simulink model "sampleModel1670"  (R2023a)
settings: Solver=VariableStepAuto  StartTime=0.0  StopTime=10.0  RelTol=1e-3
libraries: hdlsllib x7, simulink x1
settings Model: Creator=user1  LastModifiedBy=user1

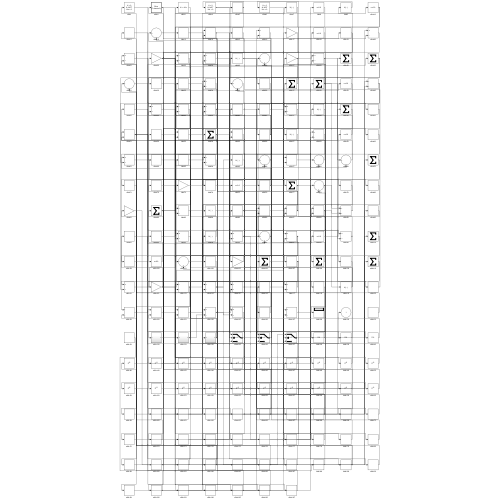
[thumbnail: Simulink's stored preview of the top-level diagram]
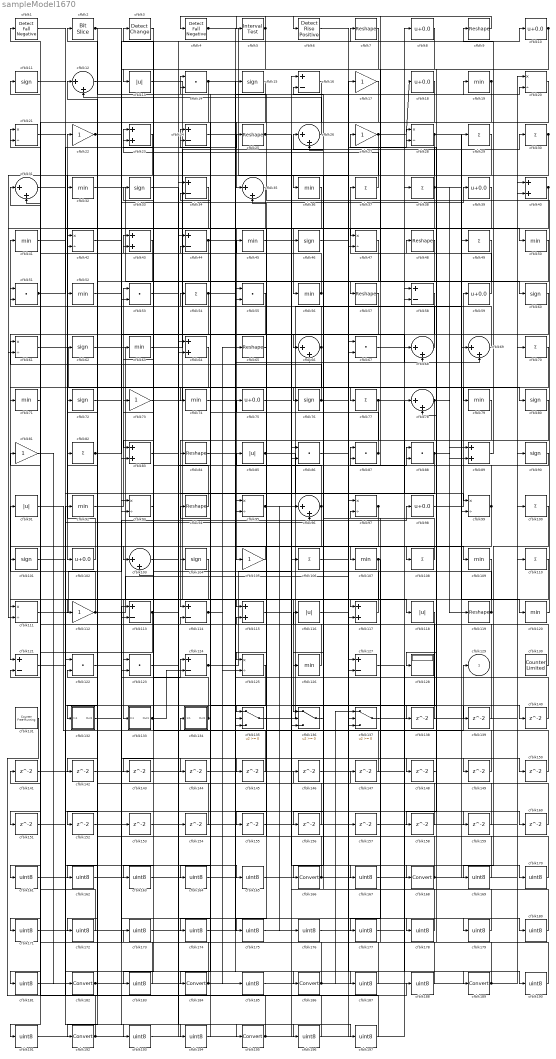
== system sampleModel1670 ==
  cfblk1 : hdlsllib/Logic and Bit Operations/Detect Fall Negative  vinit=0  OutDataTypeStr=boolean
  cfblk{8,10,18,39,59,75,98,102} (8 alike) : Bias  Bias=0.0  SaturateOnIntegerOverflow=off
  cfblk{29..30,37..38,49,54,70,77,82,100,106,108,110} (13 alike) : Sum  Inputs=+
  cfblk{11,15,33,46,60,62,72,76,80,90,101,104} (12 alike) : Signum
  cfblk{12,26,31,35,66,68..69,78,96,103} (10 alike) : Sum  Inputs=|++
  cfblk{17,22,27,73,81,105,112} (7 alike) : Gain
  cfblk{19,32,36,41,45,50,52,56,63,71,74,79,92,107,109,120,126} (17 alike) : MinMax
  cfblk{20..21,28,42,47,61,93,95,97,99,111,125} (12 alike) : Product  Inputs=*/  RndMeth=Zero  SaturateOnIntegerOverflow=on
  cfblk{16,24,34,44,58,113..114,121,124,127} (10 alike) : Sum  Inputs=+-
  cfblk{23,40,43,64,83,89,115,117} (8 alike) : Sum
  cfblk{13,85,91,116,118} (5 alike) : Abs  SaturateOnIntegerOverflow=off
  cfblk{7,9,25,48,57,65,84,94,119} (9 alike) : Reshape
  cfblk{14,51,53,55,67,86..88,122..123} (10 alike) : DotProduct  OutDataTypeStr=Inherit: Inherit via internal rule
  cfblk128 : Display
  cfblk130 : hdlsllib/Sources/Counter Limited  uplimit=7  tsamp=-1
  cfblk131 : hdlsllib/Sources/Counter Free-Running  NumBits=16  tsamp=-1
  cfblk132 : Subsystem
      settings: LibrarySourceBlock=|
      | hdlsllib/Ports &
      | Subsystems/Subsystem
  cfblk133 : Subsystem
      settings: LibrarySourceBlock=|
      | hdlsllib/Ports &
      | Subsystems/Subsystem
  cfblk134 : Subsystem
      settings: LibrarySourceBlock=|
      | hdlsllib/Ports &
      | Subsystems/Subsystem
  cfblk135 : Switch  SaturateOnIntegerOverflow=off  InputSameDT=off
  cfblk136 : Switch  SaturateOnIntegerOverflow=off  InputSameDT=off
  cfblk137 : Switch  SaturateOnIntegerOverflow=off  InputSameDT=off
  cfblk{138..160} (23 alike) : Delay  SampleTime=1
  cfblk{161..165,167,169..181,183,185,187..188,190..191,193..194,196..197} (29 alike) : DataTypeConversion  OutDataTypeStr=uint8  SaturateOnIntegerOverflow=off  RndMeth=Floor
  cfblk{166,168,182,184,186,189,192,195} (8 alike) : DataTypeConversion  SaturateOnIntegerOverflow=off  RndMeth=Floor
  cfblk2 : hdlsllib/Logic and Bit Operations/Bit Slice  lidx=7  ridx=0
  cfblk3 : simulink/Logic and Bit Operations/Detect Change  vinit=0  OutDataTypeStr=boolean
      settings: LibrarySourceBlock=|
      | hdlsllib/Logic and Bit
      | Operations/Detect
      | Change
  cfblk4 : hdlsllib/Logic and Bit Operations/Detect Fall Negative  vinit=0  OutDataTypeStr=boolean
  cfblk5 : hdlsllib/Logic and Bit Operations/Interval Test  IntervalClosedRight=on  uplimit=0.5  IntervalClosedLeft=on  lowlimit=-0.5  OutDataTypeStr=boolean
  cfblk6 : hdlsllib/Logic and Bit Operations/Detect Rise Positive  vinit=0  OutDataTypeStr=boolean
  cfblk129 : Outport  VectorParamsAs1DForOutWhenUnconnected=off
  wires:
  cfblk114/1 -> cfblk65/1, cfblk185/1
  cfblk68/1 -> cfblk22/1
  cfblk77/1 -> cfblk114/1, cfblk99/1
  cfblk7/1 -> cfblk13/1
  cfblk38/1 -> cfblk6/1, cfblk119/1, cfblk36/1, cfblk60/1, cfblk156/1
  cfblk120/1 -> cfblk2/1
  cfblk85/1 -> cfblk137/2, cfblk167/1
  cfblk49/1 -> cfblk121/1
  cfblk23/1 -> cfblk102/1
  cfblk92/1 -> cfblk53/1
  cfblk62/1 -> cfblk118/1
  cfblk63/1 -> cfblk30/1
  cfblk135/1 -> cfblk88/1
  cfblk35/1 -> cfblk105/1
  cfblk13/1 -> cfblk117/1
  cfblk20/1 -> cfblk42/1
  cfblk34/1 -> cfblk192/1
  cfblk39/1 -> cfblk56/1
  cfblk61/1 -> cfblk80/1
  cfblk48/1 -> cfblk53/2
  cfblk102/1 -> cfblk52/1
  cfblk47/1 -> cfblk132/1(In1)
  cfblk122/1 -> cfblk195/1
  cfblk110/1 -> cfblk184/1
  cfblk119/1 -> cfblk85/1, cfblk33/1
  cfblk73/1 -> cfblk77/1
  cfblk91/1 -> cfblk129/1
  cfblk98/1 -> cfblk59/1
  cfblk3/1 -> cfblk83/1
  cfblk15/1 -> cfblk35/1
  cfblk124/1 -> cfblk46/1, cfblk125/2
  cfblk95/1 -> cfblk29/1, cfblk176/1
  cfblk97/1 -> cfblk151/1, cfblk152/1
  cfblk54/1 -> cfblk71/1, cfblk137/3
  cfblk78/1 -> cfblk84/1, cfblk89/1
  cfblk44/1 -> cfblk62/1, cfblk69/2, cfblk24/1
  cfblk130/1 -> cfblk54/1
  cfblk113/1 -> cfblk87/1, cfblk171/1
  cfblk51/1 -> cfblk25/1, cfblk93/2, cfblk21/2, cfblk159/1
  cfblk31/1 -> cfblk186/1
  cfblk84/1 -> cfblk19/1
  cfblk101/1 -> cfblk115/1
  cfblk99/1 -> cfblk27/1, cfblk135/3
  cfblk65/1 -> cfblk125/1
  cfblk105/1 -> cfblk103/1
  cfblk5/1 -> cfblk4/1, cfblk163/1
  cfblk69/1 -> cfblk41/1
  cfblk111/1 -> cfblk98/1
  cfblk87/1 -> cfblk14/1, cfblk14/2
  cfblk29/1 -> cfblk76/1
  cfblk112/1 -> cfblk91/1, cfblk47/2, cfblk179/1
  cfblk107/1 -> cfblk133/1(In1), cfblk177/1
  cfblk12/1 -> cfblk79/1
  cfblk75/1 -> cfblk109/1
  cfblk66/1 -> cfblk83/2, cfblk23/2
  cfblk2/1 -> cfblk68/2, cfblk142/1
  cfblk80/1 -> cfblk108/1
  cfblk76/1 -> cfblk20/2, cfblk61/1
  cfblk16/1 -> cfblk101/1
  cfblk82/1 -> cfblk39/1, cfblk10/1
  cfblk96/1 -> cfblk123/1, cfblk75/1
  cfblk27/1 -> cfblk18/1, cfblk61/2
  cfblk53/1 -> cfblk7/1
  cfblk86/1 -> cfblk28/1
  cfblk4/1 -> cfblk97/1, cfblk117/2
  cfblk109/1 -> cfblk136/1
  cfblk123/1 -> cfblk44/1
  cfblk118/1 -> cfblk136/2
  cfblk70/1 -> cfblk166/1
  cfblk28/1 -> cfblk120/1, cfblk135/2
  cfblk30/1 -> cfblk128/1, cfblk32/1
  cfblk74/1 -> cfblk15/1
  cfblk136/1 -> cfblk26/1
  cfblk14/1 -> cfblk107/1, cfblk162/1
  cfblk19/1 -> cfblk74/1, cfblk138/1
  cfblk59/1 -> cfblk37/1
  cfblk126/1 -> cfblk21/1
  cfblk56/1 -> cfblk11/1, cfblk24/2
  cfblk94/1 -> cfblk63/1
  cfblk89/1 -> cfblk9/1
  cfblk43/1 -> cfblk112/1
  cfblk71/1 -> cfblk111/1
  cfblk121/1 -> cfblk92/1
  cfblk9/1 -> cfblk5/1
  cfblk8/1 -> cfblk57/1
  cfblk127/1 -> cfblk189/1
  cfblk50/1 -> cfblk126/1
  cfblk134/1(Out1) -> cfblk3/1, cfblk73/1
  cfblk21/1 -> cfblk47/1
  cfblk10/1 -> cfblk113/2, cfblk158/1
  cfblk37/1 -> cfblk23/1
  cfblk11/1 -> cfblk135/1
  cfblk32/1 -> cfblk69/1
  cfblk22/1 -> cfblk93/1, cfblk99/2, cfblk144/1, cfblk145/1
  cfblk137/1 -> cfblk100/1
  cfblk26/1 -> cfblk12/2
  cfblk108/1 -> cfblk51/1
  cfblk1/1 -> cfblk96/2
  cfblk117/1 -> cfblk16/2
  cfblk81/1 -> cfblk182/1
  cfblk45/1 -> cfblk168/1
  cfblk88/1 -> cfblk104/1, cfblk89/2
  cfblk133/1(Out1) -> cfblk43/1, cfblk124/2
  cfblk67/1 -> cfblk38/1
  cfblk90/1 -> cfblk87/2
  cfblk25/1 -> cfblk50/1, cfblk160/1
  cfblk132/1(Out1) -> cfblk124/1
  cfblk79/1 -> cfblk95/2
  cfblk40/1 -> cfblk66/1, cfblk111/2
  cfblk57/1 -> cfblk67/2
  cfblk138/1 -> cfblk1/1
  cfblk83/1 -> cfblk139/1
  cfblk139/1 -> cfblk78/2
  cfblk115/1 -> cfblk140/1
  cfblk140/1 -> cfblk95/1
  cfblk141/1 -> cfblk123/2
  cfblk142/1 -> cfblk96/1
  cfblk93/1 -> cfblk143/1
  cfblk144/1 -> cfblk68/1
  cfblk145/1 -> cfblk103/2
  cfblk147/1 -> cfblk43/2
  cfblk6/1 -> cfblk148/1
  cfblk148/1 -> cfblk28/2
  cfblk116/1 -> cfblk149/1
  cfblk149/1 -> cfblk26/2
  cfblk72/1 -> cfblk150/1
  cfblk150/1 -> cfblk67/1
  cfblk152/1 -> cfblk136/3
  cfblk52/1 -> cfblk153/1
  cfblk153/1 -> cfblk40/1
  cfblk33/1 -> cfblk154/1
  cfblk154/1 -> cfblk12/1
  cfblk36/1 -> cfblk155/1
  cfblk155/1 -> cfblk20/1
  cfblk156/1 -> cfblk35/2
  cfblk158/1 -> cfblk42/2
  cfblk159/1 -> cfblk114/2
  cfblk160/1 -> cfblk44/2
  cfblk64/1 -> cfblk161/1
  cfblk161/1 -> cfblk49/1
  cfblk162/1 -> cfblk64/1
  cfblk163/1 -> cfblk64/2
  cfblk17/1 -> cfblk164/1
  cfblk164/1 -> cfblk40/2
  cfblk41/1 -> cfblk165/1
  cfblk165/1 -> cfblk17/1
  cfblk166/1 -> cfblk72/1, cfblk116/1
  cfblk167/1 -> cfblk70/1
  cfblk168/1 -> cfblk94/1, cfblk115/2, cfblk97/2
  cfblk100/1 -> cfblk169/1
  cfblk169/1 -> cfblk45/1
  cfblk106/1 -> cfblk170/1
  cfblk170/1 -> cfblk16/1
  cfblk171/1 -> cfblk106/1
  cfblk55/1 -> cfblk172/1
  cfblk172/1 -> cfblk121/2
  cfblk173/1 -> cfblk55/1
  cfblk125/1 -> cfblk174/1
  cfblk174/1 -> cfblk55/2
  cfblk58/1 -> cfblk175/1
  cfblk175/1 -> cfblk8/1
  cfblk176/1 -> cfblk58/1
  cfblk177/1 -> cfblk58/2
  cfblk146/1 -> cfblk178/1
  cfblk178/1 -> cfblk86/1
  cfblk179/1 -> cfblk146/1
  cfblk157/1 -> cfblk180/1
  cfblk180/1 -> cfblk88/2
  cfblk104/1 -> cfblk181/1
  cfblk181/1 -> cfblk157/1
  cfblk182/1 -> cfblk82/1, cfblk90/1
  cfblk18/1 -> cfblk183/1
  cfblk183/1 -> cfblk81/1
  cfblk184/1 -> cfblk173/1, cfblk141/1, cfblk86/2
  cfblk185/1 -> cfblk110/1
  cfblk186/1 -> cfblk113/1, cfblk137/1
  cfblk24/1 -> cfblk187/1
  cfblk187/1 -> cfblk31/1
  cfblk131/1 -> cfblk188/1
  cfblk188/1 -> cfblk31/2
  cfblk189/1 -> cfblk147/1, cfblk48/1
  cfblk46/1 -> cfblk190/1
  cfblk190/1 -> cfblk127/1
  cfblk60/1 -> cfblk191/1
  cfblk191/1 -> cfblk127/2
  cfblk192/1 -> cfblk51/2, cfblk78/1
  cfblk151/1 -> cfblk193/1
  cfblk193/1 -> cfblk34/1
  cfblk42/1 -> cfblk194/1
  cfblk194/1 -> cfblk34/2
  cfblk195/1 -> cfblk66/2, cfblk134/1(In1)
  cfblk103/1 -> cfblk196/1
  cfblk196/1 -> cfblk122/1
  cfblk143/1 -> cfblk197/1
  cfblk197/1 -> cfblk122/2

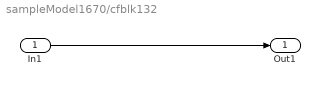
== system sampleModel1670/cfblk132 ==
  In1 : Inport
  Out1 : Outport
  wires:
  In1/1 -> Out1/1

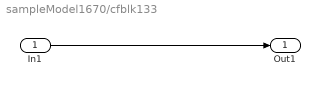
== system sampleModel1670/cfblk133 ==
  In1 : Inport
  Out1 : Outport
  wires:
  In1/1 -> Out1/1

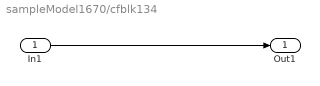
== system sampleModel1670/cfblk134 ==
  In1 : Inport
  Out1 : Outport
  wires:
  In1/1 -> Out1/1
